simulink model "testing_backlash"  (R2017a)
settings: Solver=FixedStepAuto  StartTime=0.0  StopTime=10.0  FixedStep=0.01  RelTol=1e-3
settings Model: Creator=Henry  LastModifiedBy=Henry

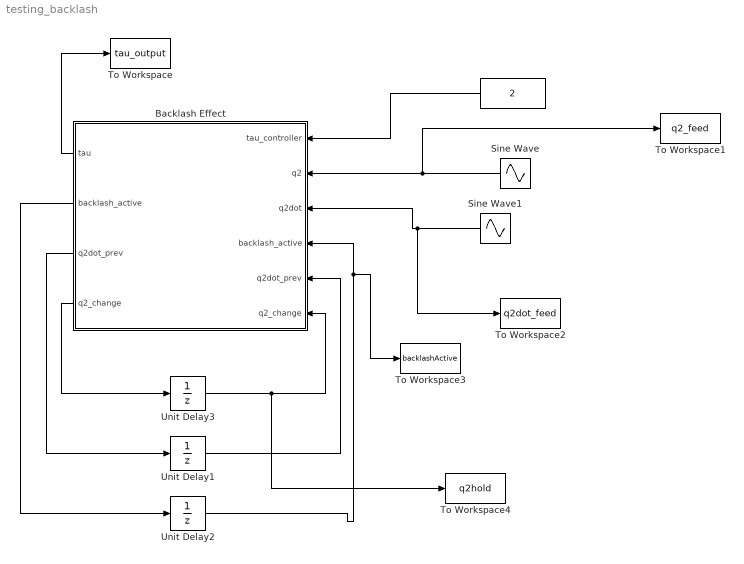
== system testing_backlash ==
  " " : Constant  Value=2
  Backlash Effect : MATLAB Function  TreatAsAtomicUnit=on
  Sine Wave : Sin  Frequency=3.6  SampleTime=0
  Sine Wave1 : Sin  Frequency=3.6  Phase=pi/2  SampleTime=0
  To Workspace : ToWorkspace  VariableName=tau_output  SaveFormat=Timeseries  SampleTime=-1
  To Workspace1 : ToWorkspace  VariableName=q2_feed  SaveFormat=Timeseries  SampleTime=-1
  To Workspace2 : ToWorkspace  VariableName=q2dot_feed  SaveFormat=Timeseries  SampleTime=-1
  To Workspace3 : ToWorkspace  VariableName=backlashActive  SaveFormat=Timeseries  SampleTime=-1
  To Workspace4 : ToWorkspace  VariableName=q2hold  SaveFormat=Timeseries  SampleTime=-1
  Unit Delay1 : UnitDelay  SampleTime=-1
  Unit Delay2 : UnitDelay  SampleTime=-1
  Unit Delay3 : UnitDelay  SampleTime=-1
  wires:
  Unit Delay2/1 -> To Workspace3/1, Backlash Effect/4("backlash_active ")
  Backlash Effect/4(q2_change) -> Unit Delay3/1
  Unit Delay3/1 -> To Workspace4/1, Backlash Effect/6("q2_change ")
  Backlash Effect/2(backlash_active) -> Unit Delay2/1
  Unit Delay1/1 -> Backlash Effect/5("q2dot_prev ")
  Backlash Effect/3(q2dot_prev) -> Unit Delay1/1
  " "/1 -> Backlash Effect/1(tau_controller)
  Sine Wave/1 -> To Workspace1/1, Backlash Effect/2(q2)
  Sine Wave1/1 -> To Workspace2/1, Backlash Effect/3(q2dot)
  Backlash Effect/1(tau) -> To Workspace/1

== matlab function testing_backlash/Backlash Effect ==
  data: tau_controller input; q2 input; q2dot input; tau output; backlash_active input; q2dot_prev input; backlash_active output; q2dot_prev output; q2_change input; q2_change output
function [tau,backlash_active,q2dot_prev,q2_change] = gearbox_backlash_test(tau_controller,q2,q2dot,backlash_active,q2dot_prev,q2_change)

tau = tau_controller;
backlash_constant = 0.1;    % [rad]



if (q2dot > 0 && q2dot_prev < 0)
    backlash_active = 1;
    q2_change = q2;
    tau = -2;
end

if (q2dot < 0 && q2dot_prev > 0)
    backlash_active = -1;
    q2_change = q2;
    tau = -2;
end

if ( (backlash_active == -1 && q2 > (q2_change + backlash_active*backlash_constant)) || (backlash_active == 1 && q2 < (q2_change + backlash_active*backlash_constant)) )
    tau = -2;
else
    backlash_active = 0;
    tau = tau_controller;
    
end
q2dot_prev = q2dot;
